simulink model "ES200A_CurrMeas"  (R2013b)
settings: Solver=FixedStepDiscrete  SolverMode=SingleTasking  StartTime=0.0  StopTime=1  FixedStep=0.000125  RelTol=1e-3
values from neighbouring files (symbols this model uses):
  ARCHGLBPRM_2PI_ULS_F32 = DataDict.Constant    [ES200A_CurrMeas_DataDict.m]
  CurrMeasEolGainMax = DataDict.Calibration    [ES200A_CurrMeas_DataDict.m]
  CurrMeasEolGainMin = DataDict.Calibration    [ES200A_CurrMeas_DataDict.m]
  CurrMeasEolGainNrOfSample = DataDict.Calibration    [ES200A_CurrMeas_DataDict.m]
  CurrMeasEolGainNumer = DataDict.Calibration    [ES200A_CurrMeas_DataDict.m]
  CurrMeasEolMaxMotVel = DataDict.Calibration    [ES200A_CurrMeas_DataDict.m]
  CurrMeasEolOffsHiBrdgVltgMin = DataDict.Calibration    [ES200A_CurrMeas_DataDict.m]
  CurrMeasEolOffsHiCmuOffs = DataDict.Calibration    [ES200A_CurrMeas_DataDict.m]
  CurrMeasEolOffsLoCmuOffs = DataDict.Calibration    [ES200A_CurrMeas_DataDict.m]
  CurrMeasEolOffsMax = DataDict.Calibration    [ES200A_CurrMeas_DataDict.m]
  CurrMeasEolOffsMin = DataDict.Calibration    [ES200A_CurrMeas_DataDict.m]
  CurrMeasEolOffsNrOfSample = DataDict.Calibration    [ES200A_CurrMeas_DataDict.m]
  CurrMeasEolTranCntrThd = DataDict.Calibration    [ES200A_CurrMeas_DataDict.m]
  CurrMeasMinRqrdPhaOnTi = DataDict.Calibration    [ES200A_CurrMeas_DataDict.m]
  CurrMeasMotAgCompuDly = DataDict.Calibration    [ES200A_CurrMeas_DataDict.m]
  CurrMeasMotCurrAdcVlyWrmIninMax = DataDict.Calibration    [ES200A_CurrMeas_DataDict.m]
  CurrMeasMotCurrAdcVlyWrmIninMin = DataDict.Calibration    [ES200A_CurrMeas_DataDict.m]
  CurrMeasNtc0x05DFailStep = DataDict.Calibration    [ES200A_CurrMeas_DataDict.m]
  CurrMeasNtc0x05DPassStep = DataDict.Calibration    [ES200A_CurrMeas_DataDict.m]
  CurrMeasNtc0x06DFailStep = DataDict.Calibration    [ES200A_CurrMeas_DataDict.m]
  CurrMeasNtc0x06DPassStep = DataDict.Calibration    [ES200A_CurrMeas_DataDict.m]
  DEGREES30_MOTRAD_F32 = DataDict.Constant    [ES200A_CurrMeas_DataDict.m]
  DIFOFFSRNGCHKMAX_VOLT_F32 = DataDict.Constant    [ES200A_CurrMeas_DataDict.m]
  ELECGLBPRM_IVTRCNT_CNT_U08 = DataDict.ConfigParam    [ES200A_CurrMeas_DataDict.m]
  ELECGLBPRM_STRTUPSTCURRMEASWRMININTESTSTRT_CNT_U08 = DataDict.Constant    [ES200A_CurrMeas_DataDict.m]
  FLTINJ_CURRMEAS_MOTCURRCORRDA = DataDict.Constant    [ES200A_CurrMeas_DataDict.m]
  FLTINJ_CURRMEAS_MOTCURRCORRDD = DataDict.Constant    [ES200A_CurrMeas_DataDict.m]
  FLTINJ_CURRMEAS_TESTOK = DataDict.Constant    [ES200A_CurrMeas_DataDict.m]
  MAXCURRCORRD_AMPR_F32 = DataDict.Constant    [ES200A_CurrMeas_DataDict.m]
  PhaABCMeasdOutOfRng = DataDict.NTC    [ES200A_CurrMeas_DataDict.m]
  PhaDEFMeasOutOfRng = DataDict.NTC    [ES200A_CurrMeas_DataDict.m]
  SysGlbPrmMotPoleCnt = DataDict.ImprtdCal    [ES200A_CurrMeas_DataDict.m]
libraries: simulink x10, FixdToFloat x1
(part 2 of 7)

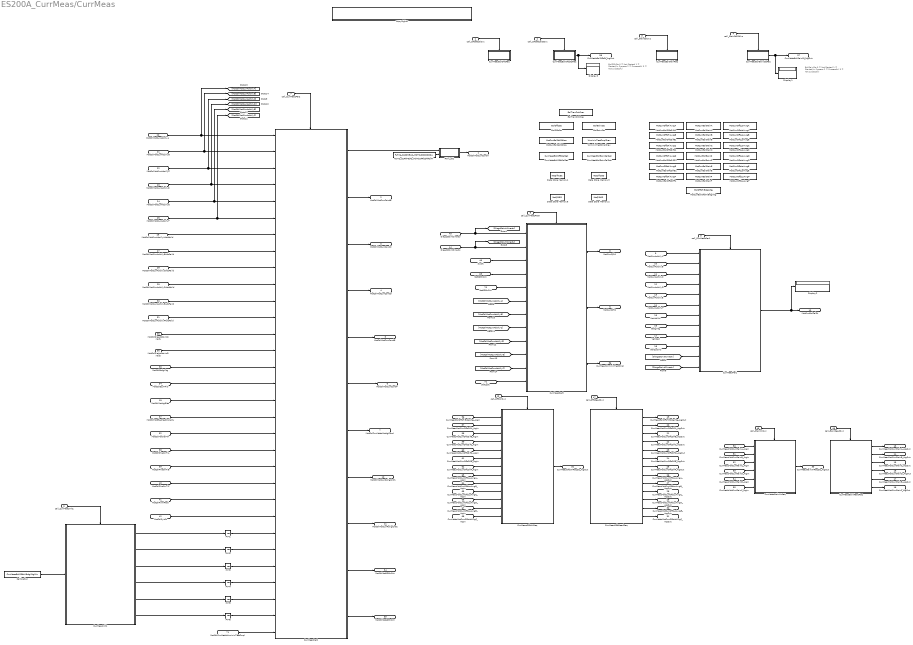
== system ES200A_CurrMeas/CurrMeas ==
  note: EolOffsSts
      | 0 = Not Started
      | 1 = Started/In Process
      | 2 = Successful
      | 3 = Not successful
  note: EolGainSts
      | 0 = Not Started
      | 1 = Started/In Process
      | 2 = Successful
      | 3 = Not successful
  call_OffsetCalSvc : Inport
  call_OffsetCalStSvc : Inport  Port=2
  call_GainCalSvc : Inport  Port=3
  call_GainCalStSvc : Inport  Port=4
  call_CurrMeasPer1 : Inport  Port=5
  call_CurrMeasInit1 : Inport  Port=6
  call_CurrMeasPer2 : Inport  Port=7
  call_CurrMeasPer3 : Inport  Port=8
  MotCurrAdcVlyA : Inport  RequirementInfo={'linktype_rmi_doors' '000089bc (/ESG Group/FDD Module Requirements/EA4 Specific/ES200A_CurrMeas)' '#ES200A_273' 'true' 'REQ: ES200A_273' '' } %GIDa_c0df36b5_bdf3_4e8f_8181_e78d75143c1c  Port=9  OutDataTypeStr=single
  MotCurrAdcVlyB : Inport  RequirementInfo={'linktype_rmi_doors' '000089bc (/ESG Group/FDD Module Requirements/EA4 Specific/ES200A_CurrMeas)' '#ES200A_274' 'true' 'REQ: ES200A_274' '' } %GIDa_0f9e2482_a92c_4bb5_9b1e_c59db09315b9  Port=10  OutDataTypeStr=single
  MotCurrAdcVlyC : Inport  RequirementInfo={'linktype_rmi_doors' '000089bc (/ESG Group/FDD Module Requirements/EA4 Specific/ES200A_CurrMeas)' '#ES200A_275' 'true' 'REQ: ES200A_275' '' } %GIDa_89f1604d_2b7d_4bdd_95c5_0defc193ca14  Port=11  OutDataTypeStr=single
  MotCurrAdcVlyD : Inport  RequirementInfo={'linktype_rmi_doors' '000089bc (/ESG Group/FDD Module Requirements/EA4 Specific/ES200A_CurrMeas)' '#ES200A_276' 'true' 'REQ: ES200A_276' '' } %GIDa_69f5d2ad_0190_4324_a10c_d70bc2b35278  Port=12  OutDataTypeStr=single
  MotCurrAdcVlyE : Inport  RequirementInfo={'linktype_rmi_doors' '000089bc (/ESG Group/FDD Module Requirements/EA4 Specific/ES200A_CurrMeas)' '#ES200A_277' 'true' 'REQ: ES200A_277' '' } %GIDa_23e7995f_a882_4818_9004_ddaffe563534  Port=13  OutDataTypeStr=single
  MotCurrAdcVlyF : Inport  RequirementInfo={'linktype_rmi_doors' '000089bc (/ESG Group/FDD Module Requirements/EA4 Specific/ES200A_CurrMeas)' '#ES200A_278' 'true' 'REQ: ES200A_278' '' } %GIDa_23433c82_0e8e_4e97_8fe7_d12880668b79  Port=14  OutDataTypeStr=single
  MotVelMrf : Inport  RequirementInfo={'linktype_rmi_doors' '000089bc (/ESG Group/FDD Module Requirements/EA4 Specific/ES200A_CurrMeas)' '#ES200A_286' 'true' 'REQ: ES200A_286' '' } %GIDa_c1b8e163_dbdd_4189_a28b_6b5291256c7b  Port=15  OutDataTypeStr=single
  BrdgVltg : Inport  RequirementInfo={'linktype_rmi_doors' '000089bc (/ESG Group/FDD Module Requirements/EA4 Specific/ES200A_CurrMeas)' '#ES200A_287' 'true' 'REQ: ES200A_287' '' } %GIDa_d608f686_0b21_4408_b34c_c21e4179a203  Port=16  OutDataTypeStr=single
  VehSpd : Inport  RequirementInfo={'linktype_rmi_doors' '000089bc (/ESG Group/FDD Module Requirements/EA4 Specific/ES200A_CurrMeas)' '#ES200A_89' 'true' 'REQ: ES200A_89' '' } %GIDa_659376f8_ed19_48de_a8d7_e76ce17ef275  Port=17
  VehSpdVld : Inport  RequirementInfo={'linktype_rmi_doors' '000089bc (/ESG Group/FDD Module Requirements/EA4 Specific/ES200A_CurrMeas)' '#ES200A_88' 'true' 'REQ: ES200A_88' '' } %GIDa_b6c314dd_ec63_43ab_bf4f_f04b07ddb0e1  Port=18
  MotCtrlMotAgElec : Inport  RequirementInfo={'linktype_rmi_doors' '000089bc (/ESG Group/FDD Module Requirements/EA4 Specific/ES200A_CurrMeas)' '#ES200A_92' 'true' 'REQ: ES200A_92' '' } %GIDa_4d7a7493_9ef8_4d81_a477_518a64b7e765  Port=19
  MotCtrlMotCurrAdcVlyA : Inport  RequirementInfo={'linktype_rmi_doors' '000089bc (/ESG Group/FDD Module Requirements/EA4 Specific/ES200A_CurrMeas)' '#ES200A_51' 'true' 'REQ: ES200A_51' '' } %GIDa_095a81c9_1782_471f_8572_7f533afe7055  Port=20
  MotCtrlMotCurrAdcVlyB : Inport  RequirementInfo={'linktype_rmi_doors' '000089bc (/ESG Group/FDD Module Requirements/EA4 Specific/ES200A_CurrMeas)' '#ES200A_52' 'true' 'REQ: ES200A_52' '' } %GIDa_1f7523be_014c_4251_bbb4_8a871a4d49c5  Port=21
  MotCtrlMotCurrAdcVlyC : Inport  RequirementInfo={'linktype_rmi_doors' '000089bc (/ESG Group/FDD Module Requirements/EA4 Specific/ES200A_CurrMeas)' '#ES200A_199' 'true' 'REQ: ES200A_199' '' } %GIDa_5fb8b3b7_c8ab_4917_9242_e4db90fb3218  Port=22
  MotCtrlMotCurrAdcVlyD : Inport  RequirementInfo={'linktype_rmi_doors' '000089bc (/ESG Group/FDD Module Requirements/EA4 Specific/ES200A_CurrMeas)' '#ES200A_198' 'true' 'REQ: ES200A_198' '' } %GIDa_6babc139_2d65_41fe_8f6b_f26a477fe7cb  Port=23
  MotCtrlMotCurrAdcVlyE : Inport  RequirementInfo={'linktype_rmi_doors' '000089bc (/ESG Group/FDD Module Requirements/EA4 Specific/ES200A_CurrMeas)' '#ES200A_197' 'true' 'REQ: ES200A_197' '' } %GIDa_832d8bbb_07ae_43d6_a6a6_97b0d1a8a188  Port=24
  MotCtrlMotCurrAdcVlyF : Inport  RequirementInfo={'linktype_rmi_doors' '000089bc (/ESG Group/FDD Module Requirements/EA4 Specific/ES200A_CurrMeas)' '#ES200A_196' 'true' 'REQ: ES200A_196' '' } %GIDa_1aebe27d_eb72_4182_bff3_a5bc4a6bc491  Port=25
  MotCtrlMotCurrAdcVlyAAdcFaild : Inport  RequirementInfo={'linktype_rmi_doors' '000089bc (/ESG Group/FDD Module Requirements/EA4 Specific/ES200A_CurrMeas)' '#ES200A_304' 'true' 'REQ: ES200A_304' '' } %GIDa_f494d58e_edd3_43ec_86aa_bd2f5c0b1e53  Port=26
  MotCtrlMotCurrAdcVlyBAdcFaild : Inport  RequirementInfo={'linktype_rmi_doors' '000089bc (/ESG Group/FDD Module Requirements/EA4 Specific/ES200A_CurrMeas)' '#ES200A_303' 'true' 'REQ: ES200A_303' '' } %GIDa_0e0f8d0a_a5ab_4b1c_8ffd_dbb8282b9bf0  Port=27
  MotCtrlMotCurrAdcVlyCAdcFaild : Inport  RequirementInfo={'linktype_rmi_doors' '000089bc (/ESG Group/FDD Module Requirements/EA4 Specific/ES200A_CurrMeas)' '#ES200A_302' 'true' 'REQ: ES200A_302' '' } %GIDa_1192528e_2d99_4b37_9499_289561c3b4a4  Port=28
  MotCtrlMotCurrAdcVlyDAdcFaild : Inport  RequirementInfo={'linktype_rmi_doors' '000089bc (/ESG Group/FDD Module Requirements/EA4 Specific/ES200A_CurrMeas)' '#ES200A_307' 'true' 'REQ: ES200A_307' '' } %GIDa_7e7b38bf_4b7b_4790_a637_fc9d5c397a00  Port=29
  MotCtrlMotCurrAdcVlyEAdcFaild : Inport  RequirementInfo={'linktype_rmi_doors' '000089bc (/ESG Group/FDD Module Requirements/EA4 Specific/ES200A_CurrMeas)' '#ES200A_306' 'true' 'REQ: ES200A_306' '' } %GIDa_6eaae959_3778_4f9e_9310_d0c7971f3c8a  Port=30
  MotCtrlMotCurrAdcVlyFAdcFaild : Inport  RequirementInfo={'linktype_rmi_doors' '000089bc (/ESG Group/FDD Module Requirements/EA4 Specific/ES200A_CurrMeas)' '#ES200A_305' 'true' 'REQ: ES200A_305' '' } %GIDa_8855bb01_20de_4587_a0e4_b0052688bc23  Port=31
  MotCtrlMotVelMrf : Inport  RequirementInfo={'linktype_rmi_doors' '000089bc (/ESG Group/FDD Module Requirements/EA4 Specific/ES200A_CurrMeas)' '#ES200A_91' 'true' 'REQ: ES200A_91' '' } %GIDa_fea102fa_fce2_4109_814b_2df3ef72f176  Port=32
  MotCtrlBrdgVltg : Inport  RequirementInfo={'linktype_rmi_doors' '000089bc (/ESG Group/FDD Module Requirements/EA4 Specific/ES200A_CurrMeas)' '#ES200A_61' 'true' 'REQ: ES200A_61' '' } %GIDa_cd5e4f33_8989_491a_80e0_8581e11631e9  Port=33
  MotCtrlEcuTFild : Inport  RequirementInfo={'linktype_rmi_doors' '000089bc (/ESG Group/FDD Module Requirements/EA4 Specific/ES200A_CurrMeas)' '#ES200A_87' 'true' 'REQ: ES200A_87' '' } %GIDa_5b85054c_ad6e_468c_aca4_404e6983dffe  Port=34
  MotCtrlDiagcStsIvtr1Inactv : Inport  RequirementInfo={'linktype_rmi_doors' '000089bc (/ESG Group/FDD Module Requirements/EA4 Specific/ES200A_CurrMeas)' '#ES200A_208' 'true' 'REQ: ES200A_208' '' } %GIDa_529e82ef_3f8d_4637_8398_5d8bf3cd26eb  Port=35
  MotCtrlDiagcStsIvtr2Inactv : Inport  RequirementInfo={'linktype_rmi_doors' '000089bc (/ESG Group/FDD Module Requirements/EA4 Specific/ES200A_CurrMeas)' '#ES200A_207' 'true' 'REQ: ES200A_207' '' } %GIDa_9e3886d9_dde0_448f_9d09_8838b1b10c86  Port=36
  MotCtrlMotElecMeclPolarity : Inport  RequirementInfo={'linktype_rmi_doors' '000089bc (/ESG Group/FDD Module Requirements/EA4 Specific/ES200A_CurrMeas)' '#ES200A_200' 'true' 'REQ: ES200A_200' '' } %GIDa_77907b8d_0ba7_4e90_8bcd_ad3fc9990f43  Port=37
  MotCtrlPhaOnTiA : Inport  RequirementInfo={'linktype_rmi_doors' '000089bc (/ESG Group/FDD Module Requirements/EA4 Specific/ES200A_CurrMeas)' '#ES200A_65' 'true' 'REQ: ES200A_65' '' } %GIDa_099e451b_caa7_42e4_b360_282c724fe78a  Port=38
  MotCtrlPhaOnTiB : Inport  RequirementInfo={'linktype_rmi_doors' '000089bc (/ESG Group/FDD Module Requirements/EA4 Specific/ES200A_CurrMeas)' '#ES200A_83' 'true' 'REQ: ES200A_83' '' } %GIDa_67a70346_52f1_4703_8d7d_ca7873152a39  Port=39
  MotCtrlPhaOnTiC : Inport  RequirementInfo={'linktype_rmi_doors' '000089bc (/ESG Group/FDD Module Requirements/EA4 Specific/ES200A_CurrMeas)' '#ES200A_84' 'true' 'REQ: ES200A_84' '' } %GIDa_068f39c8_fa14_444f_a16b_ec5404babf4e  Port=40
  MotCtrlPwmPerd : Inport  RequirementInfo={'linktype_rmi_doors' '000089bc (/ESG Group/FDD Module Requirements/EA4 Specific/ES200A_CurrMeas)' '#ES200A_201' 'true' 'REQ: ES200A_201' '' } %GIDa_bafbe9ca_4550_48fd_8399_ca3792e61e2d  Port=41
  MotCtrlSysSt : Inport  RequirementInfo={'linktype_rmi_doors' '000089bc (/ESG Group/FDD Module Requirements/EA4 Specific/ES200A_CurrMeas)' '#ES200A_86' 'true' 'REQ: ES200A_86' '' } %GIDa_ed44c421_a527_46df_809e_315a4293c71f  Port=42
  DiagcStsIvtr1Inactv : Inport  RequirementInfo={'linktype_rmi_doors' '000089bc (/ESG Group/FDD Module Requirements/EA4 Specific/ES200A_CurrMeas)' '#ES200A_288' 'true' 'REQ: ES200A_288' '' } %GIDa_bad7288c_80f6_47b4_b2bc_78bc7e6eabeb  Port=43
  DiagcStsIvtr2Inactv : Inport  RequirementInfo={'linktype_rmi_doors' '000089bc (/ESG Group/FDD Module Requirements/EA4 Specific/ES200A_CurrMeas)' '#ES200A_289' 'true' 'REQ: ES200A_289' '' } %GIDa_0970cf46_af48_4d13_9a42_3f3aa7aa1933  Port=44
  SysSt : Inport  RequirementInfo={'linktype_rmi_doors' '000089bc (/ESG Group/FDD Module Requirements/EA4 Specific/ES200A_CurrMeas)' '#ES200A_290' 'true' 'REQ: ES200A_290' '' } %GIDa_21e9adb9_0abc_4000_aa02_057b5f68b4f6  Port=45  OutDataTypeStr=single
  call_OffsWrSvc : Inport  Description=Event  Port=46
      settings: AttributesFormatString=%<Description>
  call_OffsReadSvc : Inport  Description=Event  Port=47
      settings: AttributesFormatString=%<Description>
  call_GainWrSvc : Inport  Description=Event  Port=48
      settings: AttributesFormatString=%<Description>
  call_GainReadSvc : Inport  Description=Event  Port=49
      settings: AttributesFormatString=%<Description>
  CurrMeasMotCurrGainA_ArgIn : Inport  RequirementInfo={} %GIDa_e02e9e69_78ed_4eb2_91a0_72062f054332  Port=50  OutDataTypeStr=single
  CurrMeasMotCurrGainB_ArgIn : Inport  RequirementInfo={} %GIDa_db7f26ab_9315_4b45_91de_33999b240454  Port=51  OutDataTypeStr=single
  CurrMeasMotCurrGainC_ArgIn : Inport  RequirementInfo={} %GIDa_c8ae8faf_650a_45b5_a722_08a597d856bc  Port=52  OutDataTypeStr=single
  CurrMeasMotCurrGainD_ArgIn : Inport  RequirementInfo={} %GIDa_780b0274_d388_4a92_8bbd_4b0e21410385  Port=53  OutDataTypeStr=single
  CurrMeasMotCurrGainE_ArgIn : Inport  RequirementInfo={} %GIDa_7898b6f2_620e_4f27_b56f_7c3c7f2ad999  Port=54  OutDataTypeStr=single
  CurrMeasMotCurrGainF_ArgIn : Inport  RequirementInfo={} %GIDa_606ef075_911d_49d5_9610_a018c5302de0  Port=55  OutDataTypeStr=single
  CurrMeasEolOffsHiBrdgVltg_ArgIn : Inport  RequirementInfo={} %GIDa_fa6af4f3_85ff_4bf8_a6c9_e412efeab1a8  Port=56  OutDataTypeStr=single
  CurrMeasMotCurrOffsDifA_ArgIn : Inport  RequirementInfo={} %GIDa_a580f859_620b_4bd7_94cf_c091ce97ef48  Port=57  OutDataTypeStr=single
  CurrMeasMotCurrOffsDifB_ArgIn : Inport  RequirementInfo={} %GIDa_f9ac4c1f_e4bf_4614_bc64_2ccb482c3feb  Port=58  OutDataTypeStr=single
  CurrMeasMotCurrOffsDifC_ArgIn : Inport  RequirementInfo={} %GIDa_d3a25375_e0d4_4d3d_9169_cfe95de99717  Port=59  OutDataTypeStr=single
  CurrMeasMotCurrOffsDifD_ArgIn : Inport  RequirementInfo={} %GIDa_afe10c2f_f62c_475e_b5b9_c874d72fc14a  Port=60  OutDataTypeStr=single
  CurrMeasMotCurrOffsDifE_ArgIn : Inport  RequirementInfo={} %GIDa_131f7297_6952_4660_9a3d_9238c10ae4b9  Port=61  OutDataTypeStr=single
  CurrMeasMotCurrOffsDifF_ArgIn : Inport  RequirementInfo={} %GIDa_440baff5_75d1_487b_a658_beaab6cc737b  Port=62  OutDataTypeStr=single
  CurrMeasMotCurrOffsLoAvrgA_ArgIn : Inport  RequirementInfo={} %GIDa_7cdf518b_2bf9_4c2e_8300_0470cb3b6b1d  Port=63  OutDataTypeStr=single
  CurrMeasMotCurrOffsLoAvrgB_ArgIn : Inport  RequirementInfo={} %GIDa_b4687022_ed6c_48c9_ac78_5a7d3e037191  Port=64  OutDataTypeStr=single
  CurrMeasMotCurrOffsLoAvrgC_ArgIn : Inport  RequirementInfo={} %GIDa_8a43ef91_e991_4041_a126_efe92fb64a34  Port=65  OutDataTypeStr=single
  CurrMeasMotCurrOffsLoAvrgD_ArgIn : Inport  RequirementInfo={} %GIDa_98ca3add_2acf_4323_bb7c_eef132afdb3e  Port=66  OutDataTypeStr=single
  CurrMeasMotCurrOffsLoAvrgE_ArgIn : Inport  RequirementInfo={} %GIDa_309a34ea_c3e7_4c52_b4b8_926bd11c37f9  Port=67  OutDataTypeStr=single
  CurrMeasMotCurrOffsLoAvrgF_ArgIn : Inport  RequirementInfo={} %GIDa_97c60d7a_67e5_4bb0_98a4_769f19d93611  Port=68  OutDataTypeStr=single
  Ntc5DErrCnt : Inport  RequirementInfo={'linktype_rmi_doors' '000089bc (/ESG Group/FDD Module Requirements/EA4 Specific/ES200A_CurrMeas)' '#ES200A_283' 'true' 'REQ: ES200A_283' '' } %GIDa_db3dc899_ed28_49ab_8afb_26c7b6844030  Port=69
  Ntc6DErrCnt : Inport  RequirementInfo={'linktype_rmi_doors' '000089bc (/ESG Group/FDD Module Requirements/EA4 Specific/ES200A_CurrMeas)' '#ES200A_282' 'true' 'REQ: ES200A_282' '' } %GIDa_5541b0ee_9408_4b20_819b_320959417b6b  Port=70
  MotCtrlCurrMeasWrmIninTestCmpl : Inport  RequirementInfo={'linktype_rmi_doors' '000089bc (/ESG Group/FDD Module Requirements/EA4 Specific/ES200A_CurrMeas)' '#ES200A_281' 'true' 'REQ: ES200A_281' '' } %GIDa_76d4551b_5dfa_4cb5_ac6e_147eb016cdea  Port=71
  StrtUpSt : Inport  RequirementInfo={} %GIDa_0ce71f56_275e_4048_9bfa_db0f1d52f9c1  Port=72  OutDataTypeStr=single
  Calibration : Constant  Value=CurrMeasEolOffsHiBrdgVltgMin
  CopyRight2 : Subsystem  Description=|  mask(Copyright Information){none=on}
      | Copyright info block.                                               
      |                                                                     
      | Place copyright information at the top of every subsystem in design.
      mask prompts: none "No parameters"
      mask help: Place copyright information at the top of every subsystem in design.
      mask Display:
      | NxtrConf = 'Nexteer Confidential';
      | 
      | sys = bdroot; %handle for the current model ("system")
      | first = get_param(sys,'Created');
      | first = first(end-3:end);  %year is last four digits
      | 
      | last = get_param(sys,'LastModifiedDate');
      | if isempty(last)
      |     last = datestr(now,'yyyy');
      | else
      |     last = last(end-3:end);
      | end
      | 
      | if strcmp(first,last)
      |     fprintf('%s -- Copyright %s Nexteer',NxtrConf,first)
      | else
      |     fprintf('%s -- %s%s- %s Nexteer',NxtrConf,char(169),first,last)
      | end
  CurrMeasEolGainCalSet : DataStoreMemory  RequirementInfo={} %GIDa_591de4f5_2448_480d_8ed8_43d523d607cf  DataStoreName=CurrMeasEolGainCalSet  InitialValue=[]  StateMustResolveToSignalObject=on
  CurrMeasEolGainReq : Subsystem  TreatAsAtomicUnit=on
  CurrMeasEolGainStsReq : Subsystem  TreatAsAtomicUnit=on
  CurrMeasEolOffsCalSet : DataStoreMemory  RequirementInfo={} %GIDa_b33ead4a_006d_4204_b48c_734b578e590e  DataStoreName=CurrMeasEolOffsCalSet  InitialValue=[]  StateMustResolveToSignalObject=on
  CurrMeasEolOffsReq : Subsystem  TreatAsAtomicUnit=on
  CurrMeasEolOffsStsReq : Subsystem  TreatAsAtomicUnit=on
  CurrMeasGainReadReq : Subsystem  RequirementInfo={'linktype_rmi_doors' '000089bc (/ESG Group/FDD Module Requirements/EA4 Specific/ES200A_CurrMeas)' '#ES200A_291' 'true' 'REQ: ES200A_291' '' } %GIDa_8957165b_b1b4_40e9_8dec_6827b5c09f83  TreatAsAtomicUnit=on
  CurrMeasGainWrReq : Subsystem  RequirementInfo={'linktype_rmi_doors' '000089bc (/ESG Group/FDD Module Requirements/EA4 Specific/ES200A_CurrMeas)' '#ES200A_291' 'true' 'REQ: ES200A_291' '' } %GIDa_7d8255c9_29d8_427b_b42d_2516f239f32f  TreatAsAtomicUnit=on
  CurrMeasInit1 : Subsystem
  CurrMeasOffsReadReq : Subsystem  RequirementInfo={'linktype_rmi_doors' '000089bc (/ESG Group/FDD Module Requirements/EA4 Specific/ES200A_CurrMeas)' '#ES200A_280' 'true' 'REQ: ES200A_280' '' } %GIDa_00599343_cf2b_49ef_9f21_2a644af5a598  TreatAsAtomicUnit=on
  CurrMeasOffsWrReq : Subsystem  RequirementInfo={'linktype_rmi_doors' '000089bc (/ESG Group/FDD Module Requirements/EA4 Specific/ES200A_CurrMeas)' '#ES200A_280' 'true' 'REQ: ES200A_280' '' } %GIDa_18aa9851_9869_443d_84c1_d26183b79e00  TreatAsAtomicUnit=on
  CurrMeasPer1 : Subsystem  RequirementInfo={} %GIDa_84affd99_b25a_498e_8459_c3f66b3271fb
  CurrMeasPer2 : Subsystem  RequirementInfo={'linktype_rmi_doors' '000089bc (/ESG Group/FDD Module Requirements/EA4 Specific/ES200A_CurrMeas)' '#ES200A_246' 'true' 'REQ: ES200A_246' '' } %GIDa_57a63493_5371_4d22_a543_1f8c831268fa  TreatAsAtomicUnit=on
  CurrMeasPer3 : Subsystem  RequirementInfo={} %GIDa_9b801e3e_cd20_4b56_ba7e_8ade8f05730e
  Data Store Memory1 : DataStoreMemory  DataStoreName=NtcQlfr1EC  ReadBeforeWriteMsg=warning  WriteAfterWriteMsg=warning  WriteAfterReadMsg=warning  OutDataTypeStr=uint8
      settings: AttributesFormatString=|
      | Simulation Purpose Only.
      | Do Not Code this block
      | Diagnostic Manager Owns this requirement
  Data Store Memory2 : DataStoreMemory  DataStoreName=NtcQlfr6D  ReadBeforeWriteMsg=warning  WriteAfterWriteMsg=warning  WriteAfterReadMsg=warning  OutDataTypeStr=uint8
      settings: AttributesFormatString=|
      | Simulation Purpose Only.
      | Do Not Code this block
      | Diagnostic Manager Owns this requirement
  Data Store Memory3 : DataStoreMemory  DataStoreName=NtcQlfr1ED  ReadBeforeWriteMsg=warning  WriteAfterWriteMsg=warning  WriteAfterReadMsg=warning  OutDataTypeStr=uint8
      settings: AttributesFormatString=|
      | Simulation Purpose Only.
      | Do Not Code this block
      | Diagnostic Manager Owns this requirement
  Data Store Memory6 : DataStoreMemory  DataStoreName=NtcQlfr5D  ReadBeforeWriteMsg=warning  WriteAfterWriteMsg=warning  WriteAfterReadMsg=warning  OutDataTypeStr=uint8
      settings: AttributesFormatString=|
      | Simulation Purpose Only.
      | Do Not Code this block
      | Diagnostic Manager Owns this requirement
  Display1 : Display
  Display2 : Display
  Display3 : Display
  EolGainSts : DataStoreMemory  RequirementInfo={} %GIDa_2a65076c_eca2_482a_bd3b_b6fa147e0297  DataStoreName=EolGainSts  StateMustResolveToSignalObject=on
  EolOffsSts : DataStoreMemory  RequirementInfo={} %GIDa_ac38dcd6_72cd_4627_a2e8_6cc6a471753a  DataStoreName=EolOffsSts  StateMustResolveToSignalObject=on
  EolTranCntrPrev : DataStoreMemory  RequirementInfo={} %GIDa_28ca275c_3d99_4a79_842d_acf6c8fbcbab  DataStoreName=EolTranCntrPrev  StateMustResolveToSignalObject=on
  FLTINJ_CURRMEAS_MOTCURRCORRDA7 : Constant  Value=FLTINJ_CURRMEAS_MOTCURRCORRDA
  FltInj_f32 : Subsystem  RequirementInfo={'linktype_rmi_doors' '000089bc (/ESG Group/FDD Module Requirements/EA4 Specific/ES200A_CurrMeas)' '#ES200A_267' 'true' 'REQ: ES200A_267' '' } %GIDa_1fed031f_02dc_4c88_88cc_c43ca565c7cf  TreatAsAtomicUnit=on  VariantControl=FltInj_sim  mask(Fault_Injection){}
      mask help: Fault Injection is a simulation only block for EA3 programs.
  MotCurrEolCalStPrev : DataStoreMemory  RequirementInfo={} %GIDa_86c470bd_65be_4e3b_9dc5_09f9b38a5f42  DataStoreName=MotCurrEolCalStPrev  InitialValue=[]  OutDataTypeStr=Enum: MotCurrEolCalSt2  StateMustResolveToSignalObject=on
  MotCurrEolGainA : DataStoreMemory  RequirementInfo={} %GIDa_0cdcded9_d9f5_4b70_b43a_b467e82e3b43  DataStoreName=MotCurrEolGainA  StateMustResolveToSignalObject=on
  MotCurrEolGainB : DataStoreMemory  RequirementInfo={} %GIDa_95c7681d_bd51_4e5c_814f_506511fe8c3c  DataStoreName=MotCurrEolGainB  StateMustResolveToSignalObject=on
  MotCurrEolGainC : DataStoreMemory  RequirementInfo={} %GIDa_e6247b93_05a8_4559_945c_1485f3d3451b  DataStoreName=MotCurrEolGainC  StateMustResolveToSignalObject=on
  MotCurrEolGainD : DataStoreMemory  RequirementInfo={} %GIDa_0da5824c_5efe_4cd3_a825_92f95fb02da7  DataStoreName=MotCurrEolGainD  StateMustResolveToSignalObject=on
  MotCurrEolGainE : DataStoreMemory  RequirementInfo={} %GIDa_480884d9_ef96_4da6_8691_d0b2bab861d6  DataStoreName=MotCurrEolGainE  StateMustResolveToSignalObject=on
  MotCurrEolGainF : DataStoreMemory  RequirementInfo={} %GIDa_de76fcb4_1c5b_460f_bf6c_4e8db1f87278  DataStoreName=MotCurrEolGainF  StateMustResolveToSignalObject=on
  MotCurrEolOffsDifA1 : DataStoreMemory  RequirementInfo={} %GIDa_444feee9_9f70_442f_bf9a_a9ec9180fc37  DataStoreName=MotCurrOffsHiAvrgA  StateMustResolveToSignalObject=on
  MotCurrEolOffsDifB1 : DataStoreMemory  RequirementInfo={} %GIDa_513afa24_f842_4ff3_abb9_ebc7591f1895  DataStoreName=MotCurrOffsHiAvrgB  StateMustResolveToSignalObject=on
  MotCurrEolOffsDifC1 : DataStoreMemory  RequirementInfo={} %GIDa_ab8fd377_6114_4dc8_bf24_ca9533aeef69  DataStoreName=MotCurrOffsHiAvrgC  StateMustResolveToSignalObject=on
  MotCurrEolOffsDifD1 : DataStoreMemory  RequirementInfo={} %GIDa_132a1008_e476_415b_ad4f_deeb5f08c617  DataStoreName=MotCurrOffsHiAvrgD  StateMustResolveToSignalObject=on
  MotCurrEolOffsDifE1 : DataStoreMemory  RequirementInfo={} %GIDa_5d5b1c6d_198c_4ef8_8343_bfe05d41612b  DataStoreName=MotCurrOffsHiAvrgE  StateMustResolveToSignalObject=on
  MotCurrEolOffsDifF1 : DataStoreMemory  RequirementInfo={} %GIDa_f940250a_88e7_4a50_836f_53e20d8856ce  DataStoreName=MotCurrOffsHiAvrgF  StateMustResolveToSignalObject=on
  MotCurrEolOffsHiBrdgVltg : DataStoreMemory  DataStoreName=EolOffsHiBrdgVltg  StateMustResolveToSignalObject=on
  MotCurrOffsLoAvrgA : DataStoreMemory  RequirementInfo={} %GIDa_a5f97ae6_7f25_40b4_a697_9a1052d4dc2a  DataStoreName=MotCurrOffsLoAvrgA  StateMustResolveToSignalObject=on
  MotCurrOffsLoAvrgB : DataStoreMemory  RequirementInfo={} %GIDa_89736876_ea97_4c6f_8c5e_aabd2e2e9f3b  DataStoreName=MotCurrOffsLoAvrgB  StateMustResolveToSignalObject=on
  MotCurrOffsLoAvrgC : DataStoreMemory  RequirementInfo={} %GIDa_81fb40e8_80de_428a_8aed_0beac3a3c233  DataStoreName=MotCurrOffsLoAvrgC  StateMustResolveToSignalObject=on
  MotCurrOffsLoAvrgD : DataStoreMemory  RequirementInfo={} %GIDa_29a27a9a_d64e_4160_91e8_54e5018e24f2  DataStoreName=MotCurrOffsLoAvrgD  StateMustResolveToSignalObject=on
  MotCurrOffsLoAvrgE : DataStoreMemory  RequirementInfo={} %GIDa_36f812db_a170_4432_bb07_a4319804f31a  DataStoreName=MotCurrOffsLoAvrgE  StateMustResolveToSignalObject=on
  MotCurrOffsLoAvrgF : DataStoreMemory  RequirementInfo={} %GIDa_47770435_1aa2_481e_96c5_6f418f9aaa08  DataStoreName=MotCurrOffsLoAvrgF  StateMustResolveToSignalObject=on
  PIM1 : UnitDelay  SampleTime=-1  StateName=MotCurrOffsDeltaA  StateMustResolveToSignalObject=on
      settings: AttributesFormatString=%<StateName>
  PIM2 : UnitDelay  SampleTime=-1  StateName=MotCurrOffsDeltaB  StateMustResolveToSignalObject=on
      settings: AttributesFormatString=%<StateName>
  PIM3 : UnitDelay  SampleTime=-1  StateName=MotCurrOffsDeltaC  StateMustResolveToSignalObject=on
      settings: AttributesFormatString=%<StateName>
  PIM4 : UnitDelay  SampleTime=-1  StateName=MotCurrOffsDeltaD  StateMustResolveToSignalObject=on
      settings: AttributesFormatString=%<StateName>
  PIM5 : UnitDelay  SampleTime=-1  StateName=MotCurrOffsDeltaE  StateMustResolveToSignalObject=on
      settings: AttributesFormatString=%<StateName>
  PIM6 : UnitDelay  SampleTime=-1  StateName=MotCurrOffsDeltaF  StateMustResolveToSignalObject=on
      settings: AttributesFormatString=%<StateName>
  WrmIninTestCmplPrev : DataStoreMemory  RequirementInfo={} %GIDa_1037a035_f039_417f_850f_dc3d159aeb46  DataStoreName=WrmIninTestCmplPrev  StateMustResolveToSignalObject=on
  MotCtrlMotCurrCorrdA : Outport  RequirementInfo={'linktype_rmi_doors' '000089bc (/ESG Group/FDD Module Requirements/EA4 Specific/ES200A_CurrMeas)' '#ES200A_104' 'true' 'REQ: ES200A_104' '' } %GIDa_1dff5db9_265d_4b28_bde0_72b450a93f87  OutDataTypeStr=single
  MotCtrlMotCurrCorrdB : Outport  RequirementInfo={'linktype_rmi_doors' '000089bc (/ESG Group/FDD Module Requirements/EA4 Specific/ES200A_CurrMeas)' '#ES200A_103' 'true' 'REQ: ES200A_103' '' } %GIDa_fdb01424_4fee_4430_8e17_28e543392898  Port=2
  MotCtrlMotCurrCorrdC : Outport  RequirementInfo={'linktype_rmi_doors' '000089bc (/ESG Group/FDD Module Requirements/EA4 Specific/ES200A_CurrMeas)' '#ES200A_102' 'true' 'REQ: ES200A_102' '' } %GIDa_979592cd_2176_49bf_8522_256fc2f88675  Port=3
  MotCtrlMotCurrCorrdD : Outport  RequirementInfo={'linktype_rmi_doors' '000089bc (/ESG Group/FDD Module Requirements/EA4 Specific/ES200A_CurrMeas)' '#ES200A_101' 'true' 'REQ: ES200A_101' '' } %GIDa_db5c0e22_723d_402a_8e01_d021b97c48d2  Port=4
  MotCtrlMotCurrCorrdE : Outport  RequirementInfo={'linktype_rmi_doors' '000089bc (/ESG Group/FDD Module Requirements/EA4 Specific/ES200A_CurrMeas)' '#ES200A_100' 'true' 'REQ: ES200A_100' '' } %GIDa_46066123_d136_4557_8bd3_745493383de9  Port=5
  MotCtrlMotCurrCorrdF : Outport  RequirementInfo={'linktype_rmi_doors' '000089bc (/ESG Group/FDD Module Requirements/EA4 Specific/ES200A_CurrMeas)' '#ES200A_99' 'true' 'REQ: ES200A_99' '' } %GIDa_7bf8d788_fa93_4d7e_8bb8_4b9ac969ba87  Port=6
  MotCtrlCurrMeasMotAgCorrd : Outport  RequirementInfo={'linktype_rmi_doors' '000089bc (/ESG Group/FDD Module Requirements/EA4 Specific/ES200A_CurrMeas)' '#ES200A_202' 'true' 'REQ: ES200A_202' '' } %GIDa_754d1f27_ffab_418c_9dca_d6a0b56eaec1  Port=7
  MotCurrQlfr1 : Outport  RequirementInfo={'linktype_rmi_doors' '000089bc (/ESG Group/FDD Module Requirements/EA4 Specific/ES200A_CurrMeas)' '#ES200A_97' 'true' 'REQ: ES200A_97' '' } %GIDa_18a830ca_d3a7_4d1b_9e32_4eb30b225d89  Port=8
  MotCurrQlfr2 : Outport  RequirementInfo={'linktype_rmi_doors' '000089bc (/ESG Group/FDD Module Requirements/EA4 Specific/ES200A_CurrMeas)' '#ES200A_109' 'true' 'REQ: ES200A_109' '' } %GIDa_49541905_8294_462f_8621_ed36cdfdfd3f  Port=9
  MotCtrlMotCurrRollgCntr1 : Outport  RequirementInfo={'linktype_rmi_doors' '000089bc (/ESG Group/FDD Module Requirements/EA4 Specific/ES200A_CurrMeas)' '#ES200A_95' 'true' 'REQ: ES200A_95' '' } %GIDa_ac98b500_2a18_40fe_8de9_b84d0bdaabf9  Port=10
  MotCtrlMotCurrRollgCntr2 : Outport  RequirementInfo={'linktype_rmi_doors' '000089bc (/ESG Group/FDD Module Requirements/EA4 Specific/ES200A_CurrMeas)' '#ES200A_110' 'true' 'REQ: ES200A_110' '' } %GIDa_bd1a76e4_b00a_47e8_b8b1_88fe16083247  Port=11
  MotCurrEolCalSt : Outport  RequirementInfo={} %GIDa_fd9240e7_4529_4c62_b454_348f08d6676f  Port=12
  CurrMeasMotCurrGainA_ArgOut : Outport  RequirementInfo={} %GIDa_da7a6040_633d_46e5_ae95_65ba6dec5e9f  Port=13
  CurrMeasMotCurrGainB_ArgOut : Outport  RequirementInfo={} %GIDa_d097335f_94df_4cb8_a043_f5a4f0b23977  Port=14
  CurrMeasMotCurrGainC_ArgOut : Outport  RequirementInfo={} %GIDa_67611eb2_a368_4dac_965f_f3e07cb693b0  Port=15
  CurrMeasMotCurrGainD_ArgOut : Outport  RequirementInfo={} %GIDa_e4cfea85_d2ae_4b53_b6c8_c5746416f052  Port=16
  CurrMeasMotCurrGainE_ArgOut : Outport  RequirementInfo={} %GIDa_9047f291_3bf8_41f2_997d_8122ac4288af  Port=17
  CurrMeasMotCurrGainF_ArgOut : Outport  RequirementInfo={} %GIDa_a9045a20_8629_47ad_81f3_f2d35e91d1d5  Port=18
  CurrMeasEolOffsHiBrdgVltg_ArgOut : Outport  RequirementInfo={} %GIDa_6f14f073_fb34_4356_a251_3e2812a35cf6  Port=19
  CurrMeasMotCurrOffsDifA_ArgOut : Outport  RequirementInfo={} %GIDa_6978b6dc_dfec_4ba5_973e_c8055ea8aa8e  Port=20
  CurrMeasMotCurrOffsDifB_ArgOut : Outport  RequirementInfo={} %GIDa_56fe9afb_6bc1_407e_99ef_4392c36577ae  Port=21
  CurrMeasMotCurrOffsDifC_ArgOut : Outport  RequirementInfo={} %GIDa_e712ffdc_46d2_4e6f_9650_1a27a675428a  Port=22
  CurrMeasMotCurrOffsDifD_ArgOut : Outport  RequirementInfo={} %GIDa_1a7b1c70_dc34_44b0_96eb_2e3478d281cf  Port=23
  CurrMeasMotCurrOffsDifE_ArgOut : Outport  RequirementInfo={} %GIDa_c6e139dc_3095_419c_bd17_d8187407efa4  Port=24
  CurrMeasMotCurrOffsDifF_ArgOut : Outport  RequirementInfo={} %GIDa_debd7513_6352_4a35_b41f_74398a6d5d3c  Port=25
  CurrMeasMotCurrOffsLoAvrgA_ArgOut : Outport  RequirementInfo={} %GIDa_ba2c2475_9827_4834_893e_5379a3e00aae  Port=26
  CurrMeasMotCurrOffsLoAvrgB_ArgOut : Outport  RequirementInfo={} %GIDa_333a0563_5c90_4913_bc84_87fd2f7af8f2  Port=27
  CurrMeasMotCurrOffsLoAvrgC_ArgOut : Outport  RequirementInfo={} %GIDa_e2d8bb5b_982b_4982_832a_75dd1079e656  Port=28
  CurrMeasMotCurrOffsLoAvrgD_ArgOut : Outport  RequirementInfo={} %GIDa_bd9d4bb2_bfad_44e5_a81f_bf4b3d451d64  Port=29
  CurrMeasMotCurrOffsLoAvrgE_ArgOut : Outport  RequirementInfo={} %GIDa_15455f14_b8ea_4cbd_b6e1_54f140babe3d  Port=30
  CurrMeasMotCurrOffsLoAvrgF_ArgOut : Outport  RequirementInfo={} %GIDa_75fb28ba_e3b5_475f_bef7_b44813b76bea  Port=31
  CurrMeasOffsWrReqSts_ArgOut : Outport  RequirementInfo={} %GIDa_380f915f_848d_4dec_ac44_277bb7354060  Port=32
  CurrMeasGainWrReqSts_ArgOut : Outport  RequirementInfo={} %GIDa_84786072_6eef_412a_b2e4_0317e7709056  Port=33
  MotCtrlNtc5DErrCnt : Outport  RequirementInfo={'linktype_rmi_doors' '000089bc (/ESG Group/FDD Module Requirements/EA4 Specific/ES200A_CurrMeas)' '#ES200A_284' 'true' 'REQ: ES200A_284' '' } %GIDa_074f5aec_b232_416b_9243_92a813652c29  Port=34
  MotCtrlNtc6DErrCnt : Outport  RequirementInfo={'linktype_rmi_doors' '000089bc (/ESG Group/FDD Module Requirements/EA4 Specific/ES200A_CurrMeas)' '#ES200A_285' 'true' 'REQ: ES200A_285' '' } %GIDa_fc9f5cfb_0901_4a5f_b539_049481569970  Port=35
  CurrMeasWrmIninTestCmpl : Outport  RequirementInfo={'linktype_rmi_doors' '000089bc (/ESG Group/FDD Module Requirements/EA4 Specific/ES200A_CurrMeas)' '#ES200A_204' 'true' 'REQ: ES200A_204' '' } %GIDa_5f26b73d_e8be_4948_a5a9_78d6c253a6a7  Port=36
  CurrMeasEolGainSt_ArgOut : Outport  RequirementInfo={'linktype_rmi_doors' '000089bc (/ESG Group/FDD Module Requirements/EA4 Specific/ES200A_CurrMeas)' '#ES200A_104' 'true' 'REQ: ES200A_104' '' } %GIDa_154fd1bd_d37b_493a_8560_1523c4a1120f  Port=37
  CurrMeasEolOffsSt_ArgOut : Outport  RequirementInfo={'linktype_rmi_doors' '000089bc (/ESG Group/FDD Module Requirements/EA4 Specific/ES200A_CurrMeas)' '#ES200A_104' 'true' 'REQ: ES200A_104' '' } %GIDa_1f2479cf_f1ca_4399_894d_03e47417324e  Port=38
  wires:
  Calibration/1 -> CurrMeasInit1/1(CurrMeasEolOffsHiBrdgVltgMin)
  call_CurrMeasPer2/1 -> CurrMeasPer2/Trigger
  call_CurrMeasInit1/1 -> CurrMeasInit1/Trigger
  call_GainCalSvc/1 -> CurrMeasEolGainReq/Trigger
  MotCtrlMotCurrAdcVlyEAdcFaild/1 -> CurrMeasPer2/11(MotCtrlMotCurrAdcVlyEAdcFaild)
  MotCtrlMotCurrAdcVlyDAdcFaild/1 -> CurrMeasPer2/10(MotCtrlMotCurrAdcVlyDAdcFaild)
  MotCtrlMotCurrAdcVlyFAdcFaild/1 -> CurrMeasPer2/12(MotCtrlMotCurrAdcVlyFAdcFaild)
  MotCtrlDiagcStsIvtr1Inactv/1 -> CurrMeasPer2/13(MotCtrlDiagcStsIvtr1Inactv)
  MotCtrlDiagcStsIvtr2Inactv/1 -> CurrMeasPer2/14(MotCtrlDiagcStsIvtr2Inactv)
  MotCtrlEcuTFild/1 -> CurrMeasPer2/16(MotCtrlEcuTFild)
  MotCtrlMotAgElec/1 -> CurrMeasPer2/17(MotCtrlMotAgElec)
  MotCtrlMotElecMeclPolarity/1 -> CurrMeasPer2/18(MotCtrlMotElecMeclPolarity)
  MotCtrlMotVelMrf/1 -> CurrMeasPer2/19(MotCtrlMotVelMrf)
  MotCtrlPwmPerd/1 -> CurrMeasPer2/23(MotCtrlPwmPerd)
  MotCtrlSysSt/1 -> CurrMeasPer2/24(MotCtrlSysSt)
  CurrMeasInit1/1(MotCurrOffsDeltaA) -> PIM1/1
  CurrMeasInit1/2(MotCurrOffsDeltaB) -> PIM2/1
  CurrMeasInit1/3(MotCurrOffsDeltaC) -> PIM3/1
  CurrMeasInit1/4(MotCurrOffsDeltaD) -> PIM4/1
  CurrMeasInit1/5(MotCurrOffsDeltaE) -> PIM5/1
  CurrMeasInit1/6(MotCurrOffsDeltaF) -> PIM6/1
  call_OffsetCalSvc/1 -> CurrMeasEolOffsReq/Trigger
  call_OffsetCalStSvc/1 -> CurrMeasEolOffsStsReq/Trigger
  call_GainCalStSvc/1 -> CurrMeasEolGainStsReq/Trigger
  CurrMeasEolOffsStsReq/1(CurrMeasEolOffsSt) -> CurrMeasEolOffsSt_ArgOut/1, Display3/1
  CurrMeasEolGainStsReq/1(CurrMeasEolGainSt) -> CurrMeasEolGainSt_ArgOut/1, Display1/1
  PIM4/1 -> CurrMeasPer2/28(MotCurrOffsDeltaD)
  PIM6/1 -> CurrMeasPer2/30(MotCurrOffsDeltaF)
  PIM5/1 -> CurrMeasPer2/29(MotCurrOffsDeltaE)
  call_CurrMeasPer1/1 -> CurrMeasPer1/Trigger
  CurrMeasPer1/1(MotCurrEolCalSt) -> MotCurrEolCalSt/1, Display2/1
  VehSpdVld/1 -> CurrMeasPer1/10(VehSpdVld)
  VehSpd/1 -> CurrMeasPer1/9(VehSpd)
  BrdgVltg/1 -> CurrMeasPer1/8(BrdgVltg)
  MotVelMrf/1 -> CurrMeasPer1/7(MotVelMrf)
  MotCtrlMotCurrAdcVlyAAdcFaild/1 -> CurrMeasPer2/7(MotCtrlMotCurrAdcVlyAAdcFaild)
  MotCtrlMotCurrAdcVlyCAdcFaild/1 -> CurrMeasPer2/9(MotCtrlMotCurrAdcVlyCAdcFaild)
  MotCtrlMotCurrAdcVlyBAdcFaild/1 -> CurrMeasPer2/8(MotCtrlMotCurrAdcVlyBAdcFaild)
  MotCtrlBrdgVltg/1 -> CurrMeasPer2/15(BrdgVltg)
  MotCtrlPhaOnTiA/1 -> CurrMeasPer2/20(MotCtrlPhaOnTiA)
  MotCtrlPhaOnTiB/1 -> CurrMeasPer2/21(MotCtrlPhaOnTiB)
  MotCtrlPhaOnTiC/1 -> CurrMeasPer2/22(MotCtrlPhaOnTiC)
  PIM1/1 -> CurrMeasPer2/25(MotCurrOffsDeltaA)
  PIM3/1 -> CurrMeasPer2/27(MotCurrOffsDeltaC)
  PIM2/1 -> CurrMeasPer2/26(MotCurrOffsDeltaB)
  call_CurrMeasPer3/1 -> CurrMeasPer3/Trigger
  DiagcStsIvtr2Inactv/1 -> [DiagcStsIvtr2Inactv], CurrMeasPer3/2(DiagcStsIvtr2Inactv)
  DiagcStsIvtr1Inactv/1 -> [DiagcStsIvtr1Inactv], CurrMeasPer3/1(DiagcStsIvtr1Inactv)
  [DiagcStsIvtr1Inactv] -> CurrMeasPer1/11(DiagcStsIvtr1Inactv)
  [DiagcStsIvtr2Inactv] -> CurrMeasPer1/12(DiagcStsIvtr2Inactv)
  CurrMeasPer2/1(MotCtrlMotCurrCorrdA) -> FltInj_f32/1(Signal_In)
  CurrMeasPer2/5(MotCtrlMotCurrCorrdE) -> MotCtrlMotCurrCorrdE/1
  CurrMeasPer2/6(MotCtrlMotCurrCorrdF) -> MotCtrlMotCurrCorrdF/1
  CurrMeasPer2/7(MotCtrlCurrMeasMotAgCorrd) -> MotCtrlCurrMeasMotAgCorrd/1
  CurrMeasPer2/8(MotCtrlMotCurrRollgCntr1) -> MotCtrlMotCurrRollgCntr1/1
  CurrMeasPer2/9(MotCtrlMotCurrRollgCntr2) -> MotCtrlMotCurrRollgCntr2/1
  CurrMeasPer2/3(MotCtrlMotCurrCorrdC) -> MotCtrlMotCurrCorrdC/1
  CurrMeasPer2/4(MotCtrlMotCurrCorrdD) -> MotCtrlMotCurrCorrdD/1
  CurrMeasPer2/2(MotCtrlMotCurrCorrdB) -> MotCtrlMotCurrCorrdB/1
  CurrMeasPer3/1(MotCurrQlfr1) -> MotCurrQlfr1/1
  CurrMeasPer3/2(MotCurrQlfr2) -> MotCurrQlfr2/1
  SysSt/1 -> CurrMeasPer3/3(SysSt)
  MotCurrAdcVlyE/1 -> CurrMeasPer1/5(MotCurrAdcVlyE)
  MotCurrAdcVlyF/1 -> CurrMeasPer1/6(MotCurrAdcVlyF)
  MotCurrAdcVlyA/1 -> CurrMeasPer1/1(MotCurrAdcVlyA)
  MotCurrAdcVlyC/1 -> CurrMeasPer1/3(MotCurrAdcVlyC)
  MotCurrAdcVlyB/1 -> CurrMeasPer1/2(MotCurrAdcVlyB)
  MotCurrAdcVlyD/1 -> CurrMeasPer1/4(MotCurrAdcVlyD)
  CurrMeasPer3/3(CurrMeasWrmIninTestCmpl) -> CurrMeasWrmIninTestCmpl/1
  FLTINJ_CURRMEAS_MOTCURRCORRDA7/1 -> FltInj_f32/2(Constant)
  FltInj_f32/1(Signal_Out) -> MotCtrlMotCurrCorrdA/1
  call_GainWrSvc/1 -> CurrMeasGainWrReq/Trigger
  call_GainReadSvc/1 -> CurrMeasGainReadReq/Trigger
  call_OffsWrSvc/1 -> CurrMeasOffsWrReq/Trigger
  call_OffsReadSvc/1 -> CurrMeasOffsReadReq/Trigger
  CurrMeasMotCurrGainD_ArgIn/1 -> CurrMeasGainWrReq/4(CurrMeasMotCurrGainD_ArgIn)
  CurrMeasMotCurrGainE_ArgIn/1 -> CurrMeasGainWrReq/5(CurrMeasMotCurrGainE_ArgIn)
  CurrMeasMotCurrGainC_ArgIn/1 -> CurrMeasGainWrReq/3(CurrMeasMotCurrGainC_ArgIn)
  CurrMeasMotCurrGainB_ArgIn/1 -> CurrMeasGainWrReq/2(CurrMeasMotCurrGainB_ArgIn)
  CurrMeasMotCurrGainF_ArgIn/1 -> CurrMeasGainWrReq/6(CurrMeasMotCurrGainF_ArgIn)
  CurrMeasMotCurrGainA_ArgIn/1 -> CurrMeasGainWrReq/1(CurrMeasMotCurrGainA_ArgIn)
  CurrMeasGainReadReq/1(CurrMeasMotCurrGainA_ArgOut) -> CurrMeasMotCurrGainA_ArgOut/1
  CurrMeasGainReadReq/2(CurrMeasMotCurrGainB_ArgOut) -> CurrMeasMotCurrGainB_ArgOut/1
  CurrMeasGainReadReq/3(CurrMeasMotCurrGainC_ArgOut) -> CurrMeasMotCurrGainC_ArgOut/1
  CurrMeasGainReadReq/4(CurrMeasMotCurrGainD_ArgOut) -> CurrMeasMotCurrGainD_ArgOut/1
  CurrMeasGainReadReq/5(CurrMeasMotCurrGainE_ArgOut) -> CurrMeasMotCurrGainE_ArgOut/1
  CurrMeasGainReadReq/6(CurrMeasMotCurrGainF_ArgOut) -> CurrMeasMotCurrGainF_ArgOut/1
  CurrMeasOffsReadReq/1(CurrMeasEolOffsHiBrdgVltg_ArgOut) -> CurrMeasEolOffsHiBrdgVltg_ArgOut/1
  CurrMeasOffsReadReq/2(CurrMeasMotCurrOffsDifA_ArgOut) -> CurrMeasMotCurrOffsDifA_ArgOut/1
  CurrMeasOffsReadReq/3(CurrMeasMotCurrOffsDifB_ArgOut) -> CurrMeasMotCurrOffsDifB_ArgOut/1
  CurrMeasOffsReadReq/4(CurrMeasMotCurrOffsDifC_ArgOut) -> CurrMeasMotCurrOffsDifC_ArgOut/1
  CurrMeasOffsReadReq/5(CurrMeasMotCurrOffsDifD_ArgOut) -> CurrMeasMotCurrOffsDifD_ArgOut/1
  CurrMeasOffsReadReq/6(CurrMeasMotCurrOffsDifE_ArgOut) -> CurrMeasMotCurrOffsDifE_ArgOut/1
  CurrMeasOffsReadReq/7(CurrMeasMotCurrOffsDifF_ArgOut) -> CurrMeasMotCurrOffsDifF_ArgOut/1
  CurrMeasOffsReadReq/8(CurrMeasMotCurrOffsLoAvrgA_ArgOut) -> CurrMeasMotCurrOffsLoAvrgA_ArgOut/1
  CurrMeasOffsReadReq/9(CurrMeasMotCurrOffsLoAvrgB_ArgOut) -> CurrMeasMotCurrOffsLoAvrgB_ArgOut/1
  CurrMeasOffsReadReq/10(CurrMeasMotCurrOffsLoAvrgC_ArgOut) -> CurrMeasMotCurrOffsLoAvrgC_ArgOut/1
  CurrMeasOffsReadReq/11(CurrMeasMotCurrOffsLoAvrgD_ArgOut) -> CurrMeasMotCurrOffsLoAvrgD_ArgOut/1
  CurrMeasOffsReadReq/12(CurrMeasMotCurrOffsLoAvrgE_ArgOut) -> CurrMeasMotCurrOffsLoAvrgE_ArgOut/1
  CurrMeasOffsReadReq/13(CurrMeasMotCurrOffsLoAvrgF_ArgOut) -> CurrMeasMotCurrOffsLoAvrgF_ArgOut/1
  MotCtrlCurrMeasWrmIninTestCmpl/1 -> CurrMeasPer2/31(" MotCtrlCurrMeasWrmIninTestCmplPrev")
  Ntc5DErrCnt/1 -> CurrMeasPer3/4(Ntc5DErrCnt)
  Ntc6DErrCnt/1 -> CurrMeasPer3/5(Ntc6DErrCnt)
  CurrMeasPer2/10(MotCtrlNtc5DErrCnt) -> MotCtrlNtc5DErrCnt/1
  CurrMeasPer2/11(MotCtrlNtc6DErrCnt) -> MotCtrlNtc6DErrCnt/1
  CurrMeasEolOffsHiBrdgVltg_ArgIn/1 -> CurrMeasOffsWrReq/1(CurrMeasEolOffsHiBrdgVltg_ArgIn)
  CurrMeasMotCurrOffsDifA_ArgIn/1 -> CurrMeasOffsWrReq/2(CurrMeasMotCurrOffsDifA_ArgIn)
  CurrMeasMotCurrOffsDifC_ArgIn/1 -> CurrMeasOffsWrReq/4(CurrMeasMotCurrOffsDifC_ArgIn)
  CurrMeasMotCurrOffsDifF_ArgIn/1 -> CurrMeasOffsWrReq/7(CurrMeasMotCurrOffsDifF_ArgIn)
  CurrMeasMotCurrOffsDifE_ArgIn/1 -> CurrMeasOffsWrReq/6(CurrMeasMotCurrOffsDifE_ArgIn)
  CurrMeasMotCurrOffsLoAvrgF_ArgIn/1 -> CurrMeasOffsWrReq/13(CurrMeasMotCurrOffsLoAvrgF_ArgIn)
  CurrMeasMotCurrOffsDifB_ArgIn/1 -> CurrMeasOffsWrReq/3(CurrMeasMotCurrOffsDifB_ArgIn)
  CurrMeasMotCurrOffsDifD_ArgIn/1 -> CurrMeasOffsWrReq/5(CurrMeasMotCurrOffsDifD_ArgIn)
  CurrMeasMotCurrOffsLoAvrgB_ArgIn/1 -> CurrMeasOffsWrReq/9(CurrMeasMotCurrOffsLoAvrgB_ArgIn)
  CurrMeasMotCurrOffsLoAvrgA_ArgIn/1 -> CurrMeasOffsWrReq/8(CurrMeasMotCurrOffsLoAvrgA_ArgIn)
  CurrMeasMotCurrOffsLoAvrgD_ArgIn/1 -> CurrMeasOffsWrReq/11(CurrMeasMotCurrOffsLoAvrgD_ArgIn)
  CurrMeasMotCurrOffsLoAvrgC_ArgIn/1 -> CurrMeasOffsWrReq/10(CurrMeasMotCurrOffsLoAvrgC_ArgIn)
  CurrMeasMotCurrOffsLoAvrgE_ArgIn/1 -> CurrMeasOffsWrReq/12(CurrMeasMotCurrOffsLoAvrgE_ArgIn)
  CurrMeasGainWrReq/1(CurrMeasGainWrReqSts) -> CurrMeasGainWrReqSts_ArgOut/1
  CurrMeasOffsWrReq/1(CurrMeasOffsWrReqSts) -> CurrMeasOffsWrReqSts_ArgOut/1
  [MotCtrlMotCurrAdcVlyF] -> CurrMeasPer3/11(MotCtrlMotCurrAdcVlyF)
  [MotCtrlMotCurrAdcVlyE] -> CurrMeasPer3/10(MotCtrlMotCurrAdcVlyE)
  [MotCtrlMotCurrAdcVlyD] -> CurrMeasPer3/9(MotCtrlMotCurrAdcVlyD)
  [MotCtrlMotCurrAdcVlyC] -> CurrMeasPer3/8(MotCtrlMotCurrAdcVlyC)
  [MotCtrlMotCurrAdcVlyB] -> CurrMeasPer3/7(MotCtrlMotCurrAdcVlyB)
  [MotCtrlMotCurrAdcVlyA] -> CurrMeasPer3/6(MotCtrlMotCurrAdcVlyA)
  MotCtrlMotCurrAdcVlyE/1 -> [MotCtrlMotCurrAdcVlyE], CurrMeasPer2/5(MotCtrlMotCurrAdcVlyE)
  MotCtrlMotCurrAdcVlyB/1 -> [MotCtrlMotCurrAdcVlyB], CurrMeasPer2/2(MotCtrlMotCurrAdcVlyB)
  MotCtrlMotCurrAdcVlyD/1 -> [MotCtrlMotCurrAdcVlyD], CurrMeasPer2/4(MotCtrlMotCurrAdcVlyD)
  MotCtrlMotCurrAdcVlyF/1 -> [MotCtrlMotCurrAdcVlyF], CurrMeasPer2/6(MotCtrlMotCurrAdcVlyF)
  MotCtrlMotCurrAdcVlyA/1 -> [MotCtrlMotCurrAdcVlyA], CurrMeasPer2/1(MotCtrlMotCurrAdcVlyA)
  MotCtrlMotCurrAdcVlyC/1 -> [MotCtrlMotCurrAdcVlyC], CurrMeasPer2/3(MotCtrlMotCurrAdcVlyC)
  StrtUpSt/1 -> CurrMeasPer3/12(StrtUpSt)

== system ES200A_CurrMeas/CurrMeas/CopyRight2 ==

== system ES200A_CurrMeas/CurrMeas/CurrMeasEolGainReq ==
  function : TriggerPort  TriggerType=function-call
  Constant : Constant  OutDataTypeStr=Inherit: Inherit via back propagation
  CopyRight2 : Subsystem  Description=|  mask(Copyright Information){none=on}
      | Copyright info block.                                               
      |                                                                     
      | Place copyright information at the top of every subsystem in design.
      mask prompts: none "No parameters"
      mask help: Place copyright information at the top of every subsystem in design.
      mask Display:
      | NxtrConf = 'Nexteer Confidential';
      | 
      | sys = bdroot; %handle for the current model ("system")
      | first = get_param(sys,'Created');
      | first = first(end-3:end);  %year is last four digits
      | 
      | last = get_param(sys,'LastModifiedDate');
      | if isempty(last)
      |     last = datestr(now,'yyyy');
      | else
      |     last = last(end-3:end);
      | end
      | 
      | if strcmp(first,last)
      |     fprintf('%s -- Copyright %s Nexteer',NxtrConf,first)
      | else
      |     fprintf('%s -- %s%s- %s Nexteer',NxtrConf,char(169),first,last)
      | end
  EolGainSts : DataStoreWrite  DataStoreName=EolGainSts
  wires:
  Constant/1 -> EolGainSts/1

== system ES200A_CurrMeas/CurrMeas/CurrMeasEolGainStsReq ==
  function : TriggerPort  TriggerType=function-call
  CopyRight2 : Subsystem  Description=|  mask(Copyright Information){none=on}
      | Copyright info block.                                               
      |                                                                     
      | Place copyright information at the top of every subsystem in design.
      mask prompts: none "No parameters"
      mask help: Place copyright information at the top of every subsystem in design.
      mask Display:
      | NxtrConf = 'Nexteer Confidential';
      | 
      | sys = bdroot; %handle for the current model ("system")
      | first = get_param(sys,'Created');
      | first = first(end-3:end);  %year is last four digits
      | 
      | last = get_param(sys,'LastModifiedDate');
      | if isempty(last)
      |     last = datestr(now,'yyyy');
      | else
      |     last = last(end-3:end);
      | end
      | 
      | if strcmp(first,last)
      |     fprintf('%s -- Copyright %s Nexteer',NxtrConf,first)
      | else
      |     fprintf('%s -- %s%s- %s Nexteer',NxtrConf,char(169),first,last)
      | end
  EolGainSts : DataStoreRead  DataStoreName=EolGainSts  DataStoreElements=EolGainSts
  CurrMeasEolGainSt : Outport
  wires:
  EolGainSts/1 -> CurrMeasEolGainSt/1

== system ES200A_CurrMeas/CurrMeas/CurrMeasEolOffsReq ==
  function : TriggerPort  TriggerType=function-call
  Constant : Constant  OutDataTypeStr=Inherit: Inherit via back propagation
  CopyRight2 : Subsystem  Description=|  mask(Copyright Information){none=on}
      | Copyright info block.                                               
      |                                                                     
      | Place copyright information at the top of every subsystem in design.
      mask prompts: none "No parameters"
      mask help: Place copyright information at the top of every subsystem in design.
      mask Display:
      | NxtrConf = 'Nexteer Confidential';
      | 
      | sys = bdroot; %handle for the current model ("system")
      | first = get_param(sys,'Created');
      | first = first(end-3:end);  %year is last four digits
      | 
      | last = get_param(sys,'LastModifiedDate');
      | if isempty(last)
      |     last = datestr(now,'yyyy');
      | else
      |     last = last(end-3:end);
      | end
      | 
      | if strcmp(first,last)
      |     fprintf('%s -- Copyright %s Nexteer',NxtrConf,first)
      | else
      |     fprintf('%s -- %s%s- %s Nexteer',NxtrConf,char(169),first,last)
      | end
  EolOffsSts : DataStoreWrite  DataStoreName=EolOffsSts
  wires:
  Constant/1 -> EolOffsSts/1
